simulink library "StateEstimation"  (R2016b)
settings: Solver=VariableStepAuto  StartTime=0.0  StopTime=10.0  RelTol=1e-3
undefined symbols (not defined in the file): accel_bias_init, accel_bias_noise_std, accel_noise_std, cassieParameters, CassieParameters, EKF_SampleTime, gyro_bias_init, gyro_bias_noise_std, gyro_noise_std, q_init, v_init
libraries: xpcutilitieslib x35, xpcrtudplib x35, dspfdesign x10, simulink x6, slrtlib x5
(part 3 of 3)

== system StateEstimation/State Estimator Sim Test/Reconstruct State/Low Pass Filter ==
  signal : Inport  Partition=on  PartitionDimension=1  PartitionWidth=1
  selector : Inport  Port=2
  For Each : ForEach  DisableCoverage=on  IndexMode=One-based
  Lowpass Filter : dspfdesign/Lowpass Filter  FilterType=FIR  DesignForMinimumOrder=on  FilterOrder=50  PassbandFrequency=1  StopbandFrequency=10  PassbandRipple=1  StopbandAttenuation=20  InheritSampleRate=off  SampleRate=2000  SimulateUsing=Code generation  roundingMode=Floor  coeffsDataTypeStr=fixdt(1,16)
  Lowpass Filter1 : dspfdesign/Lowpass Filter  FilterType=FIR  DesignForMinimumOrder=on  FilterOrder=50  PassbandFrequency=1  StopbandFrequency=5  PassbandRipple=1  StopbandAttenuation=30  InheritSampleRate=off  SampleRate=2000  SimulateUsing=Code generation  roundingMode=Floor  coeffsDataTypeStr=fixdt(1,16)
  Switch : Switch  Criteria=u2 > Threshold
  filtered_signal : Outport  ConcatenationDimension=1
  wires:
  signal/1 -> Lowpass Filter1/1, Lowpass Filter/1
  selector/1 -> Switch/2
  Switch/1 -> filtered_signal/1
  Lowpass Filter/1 -> Switch/1
  Lowpass Filter1/1 -> Switch/3

== matlab function StateEstimation/State Estimator/Parse Outputs/Parse_Outputs ==
  data: qwi output; wi output; ai output; q output; outputs input; dq output
function [qwi, wi, ai, q, dq] = Parse_Outputs(outputs)
%
% Frames:
%   W - Cassie World (inertial frame North-West-Up)
%   N - IMU World (inertial frame North-East-Down)
%   B - Body (cassie pelvis)
%   I - IMU (cassie vectorNav)
%   
%   Author: Ross Hartley 
%   Date:   11/06/2017
%

% Parse IMU Data from the VectorNav on Cassie
cassieOutputs = CassieOutputs;
cassieOutputs.setStructure(outputs);

% IMU Data
% VectorNav outputs quaternion as qin = [qw; qx; qy; qz]
qin = cassieOutputs.getVectorNavOrientation; qin = qin([2,3,4,1]); % Convert to [qx; qy; qz; qw] format
wi = cassieOutputs.getVectorNavAngularVelocity;      % {I}_\omega_{NI}   or   {I}_\omega_{WI}
ai = cassieOutputs.getVectorNavLinearAcceleration;   % {I}_a_{NI}        or   {I}_a_{WI}
Rni = Angles.Quaternion_to_Rotation(qin)'; % R_{NI}
Rbi = R_VectorNav_to_Pelvis(zeros(14,1))';    % R_{BI} 
Rwn = Angles.Rx(pi);                % R_{WN}
Rwi = Rwn*Rni;                      % R_{WI}
Rwb = Rwi*Rbi';                     % R_{WB}
qwi = Angles.Rotation_to_Quaternion(Rwi);
 
% Compute angular velocity of body frame:
%      {I}_\omega_{NI} = {I}_\omega_{NW} + {I}_\omega_{WB} + {I}_\omega_{BI}
%                      =        0        + {I}_\omega_{WB} +       0
%  =>  {B}_\omega_{WB} = R_{BI} * {I}_\omega_{NI}
wb = Rbi*wi; % {B}_\omega_{WB}

% Get positions
qq = Angles.Rotation_to_Euler(Rwb);
qaR = cassieOutputs.getRightLegMotorPositions;
qjR =  cassieOutputs.getRightLegJointPositions;
qaL = cassieOutputs.getLeftLegMotorPositions;
qjL =  cassieOutputs.getLeftLegJointPositions;

% Get velocities
dqq = Angles.AngularVelocity_to_EulerRates(qq, wb);
dqaR = cassieOutputs.getRightLegMotorVelocities;
dqjR =  cassieOutputs.getRightLegJointVelocities;
dqaL = cassieOutputs.getLeftLegMotorVelocities;
dqjL =  cassieOutputs.getLeftLegJointVelocities;

% Construct State Vector
q = [zeros(3,1); qq; qaL(1:3); qaL(4); qjL(1); qjL(2); qaL(5); qaR(1:3); qaR(4); qjR(1); qjR(2); qaR(5)];
dq = [zeros(3,1); dqq; dqaL(1:3); dqaL(4); dqjL(1); dqjL(2); dqaL(5); dqaR(1:3); dqaR(4); dqjR(1); dqjR(2); dqaR(5)];

end

== matlab function StateEstimation/State Estimator/Contact Estimator/GRF_Estimator ==
  data: q input; GRF output; contact output
function [GRF, contact] = GRF_Estimator(q)
% Estimates the ground reaction force in the body frame of the robot
%
% Fe_i = (S_i * J_i^T)^{-1} * S_i * \tau_d
%
J_pR = J_RightToeBottom([zeros(6,1); q(7:end)]);
J_pL = J_LeftToeBottom([zeros(6,1); q(7:end)]);

qs_knee_L = q(11);
qs_tarsus_L = q(10) + q(11) + q(12) - deg2rad(13);

qs_knee_R = q(18);
qs_tarsus_R = q(17) + q(18) + q(19) - deg2rad(13);

tau_L = -[1500; 1250].*[qs_knee_L + qs_tarsus_L; qs_tarsus_L];
tau_R = -[1500; 1250].*[qs_knee_R + qs_tarsus_R; qs_tarsus_R];

GRF_L = -[J_pL([1,3],11), J_pL([1,3],12)] \ tau_L;
GRF_R = -[J_pR([1,3],18), J_pR([1,3],19)] \ tau_R;
GRF = [GRF_L; GRF_R];

% Detect contact using GRF
cL = scaleFactor(GRF(2), 50, 100);
cR = scaleFactor(GRF(4), 50, 100);
contact = [cL; cR];

end

== matlab function StateEstimation/Right-Invariant EKF/Contact Estimator/GRF_Estimator ==
  data: q input; GRF output; contact output
function [GRF, contact] = GRF_Estimator(q)
% Estimates the ground reaction force in the body frame of the robot
%
% Fe_i = (S_i * J_i^T)^{-1} * S_i * \tau_d
%
J_pR = J_RightToeBottom([zeros(6,1); q(7:end)]);
J_pL = J_LeftToeBottom([zeros(6,1); q(7:end)]);

qs_knee_L = q(11);
qs_tarsus_L = q(10) + q(11) + q(12) - deg2rad(13);

qs_knee_R = q(18);
qs_tarsus_R = q(17) + q(18) + q(19) - deg2rad(13);

tau_L = -[1500; 1250].*[qs_knee_L + qs_tarsus_L; qs_tarsus_L];
tau_R = -[1500; 1250].*[qs_knee_R + qs_tarsus_R; qs_tarsus_R];

GRF_L = -[J_pL([1,3],11), J_pL([1,3],12)] \ tau_L;
GRF_R = -[J_pR([1,3],18), J_pR([1,3],19)] \ tau_R;
GRF = [GRF_L; GRF_R];

% Detect contact using GRF
cL = scaleFactor(GRF(2), 50, 100);
cR = scaleFactor(GRF(4), 50, 100);
contact = [cL; cR];

end

== matlab function StateEstimation/Right-Invariant EKF/EKF/Send Pose UDP/ConstructPoseData ==
  data: pose_data output; mu input; Sigma input
function pose_data = ConstructPoseData(mu, Sigma)
% Construct pose data for use in ROS network
% Publish everything in pelvis frame
Rwi = Angles.Quaternion_to_Rotation(mu(7:10))';

pose_data = zeros(43,1); 
pose_data(1:3) = mu(1:3) + Rwi*p_VectorNav_to_Pelvis(zeros(14,1));
pose_data(4:7) = Angles.Rotation_to_Quaternion( (Rwi * R_VectorNav_to_Pelvis(zeros(14,1)))' );

% TODO: Convert covariance of IMU pose to Body pose (Ross) 
pose_data(8:end) = reshape(Sigma([1:3,1:3],[7:9,7:9]),[],1);

end

== matlab function StateEstimation/State Estimator/Parse Outputs/Send IMU UDP/Invert Quaterion for ROS ==
  data: q input; q_inv output
function q_inv = fcn(q)
    q_inv = Angles.Rotation_to_Quaternion( Angles.Quaternion_to_Rotation(q)' );
end

== matlab function StateEstimation/Right-Invariant EKF/Kinematic Velocity Estimator/Kinematic_Velocity ==
  data: w input; e input; e_dot input; contact input; velocity output
function velocity  = Kinematic_Velocity(w, e, e_dot, contact)
% Kinematic Velocity Estimator

if contact(1) == 1
    pL = p_VectorNav_to_LeftToeBottom(e); % {I}_p_{IL}
    J_pL = J_VectorNav_to_LeftToeBottom(e);
    velocity = -J_pL(1:3,:)*e_dot - Angles.skew(w)*pL(1:3,:); % {I}_v_{WI}
elseif contact(2) == 1
    pR = p_VectorNav_to_RightToeBottom(e); % {I}_p_{IR}
    J_pR = J_VectorNav_to_RightToeBottom(e);
    velocity = -J_pR(1:3,:)*e_dot - Angles.skew(w)*pR(1:3,:); % {I}_v_{WI}
else
    velocity = zeros(3,1);
end

end

== matlab function StateEstimation/State Estimator/Reconstruct State/Construct_State ==
  data: q output; dq output; q input; dq input; w input; contact input; mu input; ekf_enabled input; velocity output; velocity_kinematic output; filter_selector output
function [q, dq, velocity, velocity_kinematic, filter_selector] = Construct_State(q, dq, w, contact, mu, ekf_enabled)
% Construct state vector and body velocity estimate using raw data and ekf
%   
%   Inputs:
%       q           - state position vector
%       dq          - state velocity vector
%       w           - angular velocity, {I}_\omega_{WI}
%       contact     - contact indicator
%       mu          - EKF state estimate
%       ekf_enabled - EKF enable flag
%
%   Outputs:
%       q                   - 
%       dq                  - 
%       velocity            - EKF body velocity, {W}_v_{WB} 
%       velocity_kinematic  - Kinematic body velocity, {B}_v_{WB} 
%       filter_selector     - used to select low pass filter type
%
%
%   Author: Ross Hartley
%   Date:   11/07/2017

%% Settings
use_ekf_position = true;
use_ekf_orientation = false;
use_ekf_velocity = false;

%% Compute kinematic velocity
e = q(7:end);
e_dot = dq(7:end);

if contact(1) == 1
    pL = p_VectorNav_to_LeftToeBottom(e); % {I}_p_{IL}
    J_pL = J_VectorNav_to_LeftToeBottom(e);
    velocity_kinematic = -J_pL(1:3,:)*e_dot - Angles.skew(w)*pL(1:3,:); % {I}_v_{WI}
elseif contact(2) == 1
    pR = p_VectorNav_to_RightToeBottom(e); % {I}_p_{IR}
    J_pR = J_VectorNav_to_RightToeBottom(e);
    velocity_kinematic = -J_pR(1:3,:)*e_dot - Angles.skew(w)*pR(1:3,:); % {I}_v_{WI}
else
    velocity_kinematic = zeros(3,1);
end

%% Reconstruct State
Rbi = R_VectorNav_to_Pelvis(e)';    % R_{BI}

% Position
if use_ekf_position && ekf_enabled
    Rwi = Angles.Quaternion_to_Rotation(mu(7:10))';
    % {W}_p_{WB} =  {W}_p_{WI} +  {W}_p_{IB}
    q(1:3) = mu(1:3) + Rwi * p_VectorNav_to_Pelvis(e); 
end
 
% Orientation
if use_ekf_orientation && ekf_enabled
    Rwi = Angles.Quaternion_to_Rotation(mu(7:10))';
    Rwb = Rwi * Rbi';
    q(4:6) = Angles.Rotation_to_Euler( Rwb );
end

% Velocity
if use_ekf_velocity && ekf_enabled
    Rwi = Angles.Quaternion_to_Rotation(mu(7:10))';
    Rwb = Rwi * Rbi';
    % {W}_v_{WB} =  {W}_v_{WI} + R_{WI} * skew({I}_w_{WI}) * {I}_p_{IB}
    dq(1:3) = mu(4:6) + Rwi * Angles.skew(w) * p_VectorNav_to_Pelvis(e); 
    % {B}_v_{WB} = R_{BW} * {W}_v_{WB}
    velocity = Rwb' * dq(1:3);
    filter_selector = 1;
else
    Rwb = Angles.Euler_to_Rotation(q(4:6));
    Rwi = Rwb * Rbi;
    % {W}_v_{WB} =  R_{WI} * {I}_v_{WI} + R_{WI} * skew({I}_w_{WI}) * {I}_p_{IB}
    dq(1:3) = Rwi * velocity_kinematic + Rwi * Angles.skew(w) * p_VectorNav_to_Pelvis(e); 
    % {B}_v_{WB} = R_{BW} * {W}_v_{WB}
    velocity = Rwb' * dq(1:3);
    filter_selector = 0;
end



end

== matlab function StateEstimation/State Estimator/Parse Outputs/Send JointState UDP/Parse_Outputs ==
  data: q_reduced output; dq_reduced output; q input; dq input
function [q_reduced, dq_reduced] = ReduceState(q, dq)
% Reduce state vector for use in ROS network

q_reduced = q(7:end);
dq_reduced = dq(7:end);

end

== matlab function StateEstimation/State Estimator/EKF/Send Pose UDP/ConstructPoseData ==
  data: pose_data output; mu input; Sigma input
function pose_data = ConstructPoseData(mu, Sigma)
% Construct pose data for use in ROS network
% Publish everything in pelvis frame
Rwi = Angles.Quaternion_to_Rotation(mu(7:10))';

pose_data = zeros(43,1); 
pose_data(1:3) = mu(1:3) + Rwi*p_VectorNav_to_Pelvis(zeros(14,1));
pose_data(4:7) = Angles.Rotation_to_Quaternion( (Rwi * R_VectorNav_to_Pelvis(zeros(14,1)))' );

% TODO: Convert covariance of IMU pose to Body pose (Ross) 
pose_data(8:end) = reshape(Sigma([1:3,1:3],[7:9,7:9]),[],1);

end

== matlab function StateEstimation/Right-Invariant EKF/Parse Outputs/Parse_Outputs ==
  data: qwi output; wi output; ai output; q output; outputs input; dq output
function [qwi, wi, ai, q, dq] = Parse_Outputs(outputs)
%
% Frames:
%   W - Cassie World (inertial frame North-West-Up)
%   N - IMU World (inertial frame North-East-Down)
%   B - Body (cassie pelvis)
%   I - IMU (cassie vectorNav)
%   
%   Author: Ross Hartley 
%   Date:   11/06/2017
%

% Parse IMU Data from the VectorNav on Cassie
cassieOutputs = CassieOutputs;
cassieOutputs.setStructure(outputs);

% IMU Data
% VectorNav outputs quaternion as qin = [qw; qx; qy; qz]
qin = cassieOutputs.getVectorNavOrientation; qin = qin([2,3,4,1]); % Convert to [qx; qy; qz; qw] format
wi = cassieOutputs.getVectorNavAngularVelocity;      % {I}_\omega_{NI}   or   {I}_\omega_{WI}
ai = cassieOutputs.getVectorNavLinearAcceleration;   % {I}_a_{NI}        or   {I}_a_{WI}
Rni = Angles.Quaternion_to_Rotation(qin)'; % R_{NI}
Rbi = R_VectorNav_to_Pelvis(zeros(14,1))';    % R_{BI} 
Rwn = Angles.Rx(pi);                % R_{WN}
Rwi = Rwn*Rni;                      % R_{WI}
Rwb = Rwi*Rbi';                     % R_{WB}
qwi = Angles.Rotation_to_Quaternion(Rwi);
 
% Compute angular velocity of body frame:
%      {I}_\omega_{NI} = {I}_\omega_{NW} + {I}_\omega_{WB} + {I}_\omega_{BI}
%                      =        0        + {I}_\omega_{WB} +       0
%  =>  {B}_\omega_{WB} = R_{BI} * {I}_\omega_{NI}
wb = Rbi*wi; % {B}_\omega_{WB}

% Get positions
qq = Angles.Rotation_to_Euler(Rwb);
qaR = cassieOutputs.getRightLegMotorPositions;
qjR =  cassieOutputs.getRightLegJointPositions;
qaL = cassieOutputs.getLeftLegMotorPositions;
qjL =  cassieOutputs.getLeftLegJointPositions;

% Get velocities
dqq = Angles.AngularVelocity_to_EulerRates(qq, wb);
dqaR = cassieOutputs.getRightLegMotorVelocities;
dqjR =  cassieOutputs.getRightLegJointVelocities;
dqaL = cassieOutputs.getLeftLegMotorVelocities;
dqjL =  cassieOutputs.getLeftLegJointVelocities;

% Construct State Vector
q = [zeros(3,1); qq; qaL(1:3); qaL(4); qjL(1); qjL(2); qaL(5); qaR(1:3); qaR(4); qjR(1); qjR(2); qaR(5)];
dq = [zeros(3,1); dqq; dqaL(1:3); dqaL(4); dqjL(1); dqjL(2); dqaL(5); dqaR(1:3); dqaR(4); dqjR(1); dqjR(2); dqaR(5)];

end

== matlab function StateEstimation/State Estimator Sim Test/Contact Estimator/GRF_Estimator ==
  data: q input; GRF output; contact output
function [GRF, contact] = GRF_Estimator(q)
% Estimates the ground reaction force in the body frame of the robot
%
% Fe_i = (S_i * J_i^T)^{-1} * S_i * \tau_d
%
J_pR = J_RightToeBottom([zeros(6,1); q(7:end)]);
J_pL = J_LeftToeBottom([zeros(6,1); q(7:end)]);

qs_knee_L = q(11);
qs_tarsus_L = q(10) + q(11) + q(12) - deg2rad(13);

qs_knee_R = q(18);
qs_tarsus_R = q(17) + q(18) + q(19) - deg2rad(13);

tau_L = -[1500; 1250].*[qs_knee_L + qs_tarsus_L; qs_tarsus_L];
tau_R = -[1500; 1250].*[qs_knee_R + qs_tarsus_R; qs_tarsus_R];

GRF_L = -[J_pL([1,3],11), J_pL([1,3],12)] \ tau_L;
GRF_R = -[J_pR([1,3],18), J_pR([1,3],19)] \ tau_R;
GRF = [GRF_L; GRF_R];

% Detect contact using GRF
cL = scaleFactor(GRF(2), 50, 100);
cR = scaleFactor(GRF(4), 50, 100);
contact = [cL; cR];

end

== matlab function StateEstimation/Right-Invariant EKF/Parse Outputs/Send IMU UDP/Invert Quaterion for ROS ==
  data: q input; q_inv output
function q_inv = fcn(q)
    q_inv = Angles.Rotation_to_Quaternion( Angles.Quaternion_to_Rotation(q)' );
end

== matlab function StateEstimation/Right-Invariant EKF/Parse Outputs/Send JointState UDP/Parse_Outputs ==
  data: q_reduced output; dq_reduced output; q input; dq input
function [q_reduced, dq_reduced] = ReduceState(q, dq)
% Reduce state vector for use in ROS network

q_reduced = q(7:end);
dq_reduced = dq(7:end);

end

== matlab function StateEstimation/State Estimator Sim Test/EKF/Send Pose UDP/ConstructPoseData ==
  data: pose_data output; mu input; Sigma input
function pose_data = ConstructPoseData(mu, Sigma)
% Construct pose data for use in ROS network
% Publish everything in pelvis frame
Rwi = Angles.Quaternion_to_Rotation(mu(7:10))';

pose_data = zeros(43,1); 
pose_data(1:3) = mu(1:3) + Rwi*p_VectorNav_to_Pelvis(zeros(14,1));
pose_data(4:7) = Angles.Rotation_to_Quaternion( (Rwi * R_VectorNav_to_Pelvis(zeros(14,1)))' );

% TODO: Convert covariance of IMU pose to Body pose (Ross) 
pose_data(8:end) = reshape(Sigma([1:3,1:3],[7:9,7:9]),[],1);

end

== matlab function StateEstimation/State Estimator Sim Test/Kinematic Velocity Estimator/Kinematic_Velocity ==
  data: w input; e input; e_dot input; contact input; velocity output
function velocity  = Kinematic_Velocity(w, e, e_dot, contact)
% Kinematic Velocity Estimator

if contact(1) == 1
    pL = p_VectorNav_to_LeftToeBottom(e); % {I}_p_{IL}
    J_pL = J_VectorNav_to_LeftToeBottom(e);
    velocity = -J_pL(1:3,:)*e_dot - Angles.skew(w)*pL(1:3,:); % {I}_v_{WI}
elseif contact(2) == 1
    pR = p_VectorNav_to_RightToeBottom(e); % {I}_p_{IR}
    J_pR = J_VectorNav_to_RightToeBottom(e);
    velocity = -J_pR(1:3,:)*e_dot - Angles.skew(w)*pR(1:3,:); % {I}_v_{WI}
else
    velocity = zeros(3,1);
end

end

== matlab function StateEstimation/State Estimator Sim Test/Parse Outputs/Parse_Outputs ==
  data: qwi output; wi output; ai output; q output; outputs input; dq output
function [qwi, wi, ai, q, dq] = Parse_Outputs(outputs)
%
% Frames:
%   W - Cassie World (inertial frame North-West-Up)
%   N - IMU World (inertial frame North-East-Down)
%   B - Body (cassie pelvis)
%   I - IMU (cassie vectorNav)
%   
%   Author: Ross Hartley 
%   Date:   11/06/2017
%

% Parse IMU Data from the VectorNav on Cassie
cassieOutputs = CassieOutputs;
cassieOutputs.setStructure(outputs);

% IMU Data
% VectorNav outputs quaternion as qin = [qw; qx; qy; qz]
qin = cassieOutputs.getVectorNavOrientation; qin = qin([2,3,4,1]); % Convert to [qx; qy; qz; qw] format
wi = cassieOutputs.getVectorNavAngularVelocity;      % {I}_\omega_{NI}   or   {I}_\omega_{WI}
ai = cassieOutputs.getVectorNavLinearAcceleration;   % {I}_a_{NI}        or   {I}_a_{WI}
Rni = Angles.Quaternion_to_Rotation(qin)'; % R_{NI}
Rbi = R_VectorNav_to_Pelvis(zeros(14,1))';    % R_{BI} 
Rwn = Angles.Rx(pi);                % R_{WN}
Rwi = Rwn*Rni;                      % R_{WI}
Rwb = Rwi*Rbi';                     % R_{WB}
qwi = Angles.Rotation_to_Quaternion(Rwi);
 
% Compute angular velocity of body frame:
%      {I}_\omega_{NI} = {I}_\omega_{NW} + {I}_\omega_{WB} + {I}_\omega_{BI}
%                      =        0        + {I}_\omega_{WB} +       0
%  =>  {B}_\omega_{WB} = R_{BI} * {I}_\omega_{NI}
wb = Rbi*wi; % {B}_\omega_{WB}

% Get positions
qq = Angles.Rotation_to_Euler(Rwb);
qaR = cassieOutputs.getRightLegMotorPositions;
qjR =  cassieOutputs.getRightLegJointPositions;
qaL = cassieOutputs.getLeftLegMotorPositions;
qjL =  cassieOutputs.getLeftLegJointPositions;

% Get velocities
dqq = Angles.AngularVelocity_to_EulerRates(qq, wb);
dqaR = cassieOutputs.getRightLegMotorVelocities;
dqjR =  cassieOutputs.getRightLegJointVelocities;
dqaL = cassieOutputs.getLeftLegMotorVelocities;
dqjL =  cassieOutputs.getLeftLegJointVelocities;

% Construct State Vector
q = [zeros(3,1); qq; qaL(1:3); qaL(4); qjL(1); qjL(2); qaL(5); qaR(1:3); qaR(4); qjR(1); qjR(2); qaR(5)];
dq = [zeros(3,1); dqq; dqaL(1:3); dqaL(4); dqjL(1); dqjL(2); dqaL(5); dqaR(1:3); dqaR(4); dqjR(1); dqjR(2); dqaR(5)];

end

== matlab function StateEstimation/State Estimator Sim Test/Parse Outputs/Send IMU UDP/Invert Quaterion for ROS ==
  data: q input; q_inv output
function q_inv = fcn(q)
    q_inv = Angles.Rotation_to_Quaternion( Angles.Quaternion_to_Rotation(q)' );
end

== matlab function StateEstimation/State Estimator Sim Test/Parse Outputs/Send JointState UDP/Parse_Outputs ==
  data: q_reduced output; dq_reduced output; q input; dq input
function [q_reduced, dq_reduced] = ReduceState(q, dq)
% Reduce state vector for use in ROS network

q_reduced = q(7:end);
dq_reduced = dq(7:end);

end

== matlab function StateEstimation/State Estimator/Kinematic Velocity Estimator/Kinematic_Velocity ==
  data: w input; e input; e_dot input; contact input; velocity output
function velocity  = Kinematic_Velocity(w, e, e_dot, contact)
% Kinematic Velocity Estimator

if contact(1) == 1
    pL = p_VectorNav_to_LeftToeBottom(e); % {I}_p_{IL}
    J_pL = J_VectorNav_to_LeftToeBottom(e);
    velocity = -J_pL(1:3,:)*e_dot - Angles.skew(w)*pL(1:3,:); % {I}_v_{WI}
elseif contact(2) == 1
    pR = p_VectorNav_to_RightToeBottom(e); % {I}_p_{IR}
    J_pR = J_VectorNav_to_RightToeBottom(e);
    velocity = -J_pR(1:3,:)*e_dot - Angles.skew(w)*pR(1:3,:); % {I}_v_{WI}
else
    velocity = zeros(3,1);
end

end

== matlab function StateEstimation/State Estimator Sim Test/Reconstruct State/Construct_State ==
  data: q output; dq output; q input; dq input; w input; contact input; mu input; ekf_enabled input; velocity output; velocity_kinematic output; filter_selector output
function [q, dq, velocity, velocity_kinematic, filter_selector] = Construct_State(q, dq, w, contact, mu, ekf_enabled)
% Construct state vector and body velocity estimate using raw data and ekf
%   
%   Inputs:
%       q           - state position vector
%       dq          - state velocity vector
%       w           - angular velocity, {I}_\omega_{WI}
%       contact     - contact indicator
%       mu          - EKF state estimate
%       ekf_enabled - EKF enable flag
%
%   Outputs:
%       q                   - 
%       dq                  - 
%       velocity            - EKF body velocity, {W}_v_{WB} 
%       velocity_kinematic  - Kinematic body velocity, {B}_v_{WB} 
%       filter_selector     - used to select low pass filter type
%
%
%   Author: Ross Hartley
%   Date:   11/07/2017

%% Settings
use_ekf_position = true;
use_ekf_orientation = false;
use_ekf_velocity = false;

%% Compute kinematic velocity
e = q(7:end);
e_dot = dq(7:end);

if contact(1) == 1
    pL = p_VectorNav_to_LeftToeBottom(e); % {I}_p_{IL}
    J_pL = J_VectorNav_to_LeftToeBottom(e);
    velocity_kinematic = -J_pL(1:3,:)*e_dot - Angles.skew(w)*pL(1:3,:); % {I}_v_{WI}
elseif contact(2) == 1
    pR = p_VectorNav_to_RightToeBottom(e); % {I}_p_{IR}
    J_pR = J_VectorNav_to_RightToeBottom(e);
    velocity_kinematic = -J_pR(1:3,:)*e_dot - Angles.skew(w)*pR(1:3,:); % {I}_v_{WI}
else
    velocity_kinematic = zeros(3,1);
end

%% Reconstruct State
Rbi = R_VectorNav_to_Pelvis(e)';    % R_{BI}

% Position
if use_ekf_position && ekf_enabled
    Rwi = Angles.Quaternion_to_Rotation(mu(7:10))';
    % {W}_p_{WB} =  {W}_p_{WI} +  {W}_p_{IB}
    q(1:3) = mu(1:3) + Rwi * p_VectorNav_to_Pelvis(e); 
end
 
% Orientation
if use_ekf_orientation && ekf_enabled
    Rwi = Angles.Quaternion_to_Rotation(mu(7:10))';
    Rwb = Rwi * Rbi';
    q(4:6) = Angles.Rotation_to_Euler( Rwb );
end

% Velocity
if use_ekf_velocity && ekf_enabled
    Rwi = Angles.Quaternion_to_Rotation(mu(7:10))';
    Rwb = Rwi * Rbi';
    % {W}_v_{WB} =  {W}_v_{WI} + R_{WI} * skew({I}_w_{WI}) * {I}_p_{IB}
    dq(1:3) = mu(4:6) + Rwi * Angles.skew(w) * p_VectorNav_to_Pelvis(e); 
    % {B}_v_{WB} = R_{BW} * {W}_v_{WB}
    velocity = Rwb' * dq(1:3);
    filter_selector = 1;
else
    Rwb = Angles.Euler_to_Rotation(q(4:6));
    Rwi = Rwb * Rbi;
    % {W}_v_{WB} =  R_{WI} * {I}_v_{WI} + R_{WI} * skew({I}_w_{WI}) * {I}_p_{IB}
    dq(1:3) = Rwi * velocity_kinematic + Rwi * Angles.skew(w) * p_VectorNav_to_Pelvis(e); 
    % {B}_v_{WB} = R_{BW} * {W}_v_{WB}
    velocity = Rwb' * dq(1:3);
    filter_selector = 0;
end



end

== matlab function StateEstimation/Kinematic Velocity Estimator/Kinematic_Velocity ==
  data: w input; e input; e_dot input; contact input; velocity output
function velocity  = Kinematic_Velocity(w, e, e_dot, contact)
% Kinematic Velocity Estimator

if contact(1) == 1
    pL = p_VectorNav_to_LeftToeBottom(e); % {I}_p_{IL}
    J_pL = J_VectorNav_to_LeftToeBottom(e);
    velocity = -J_pL(1:3,:)*e_dot - Angles.skew(w)*pL(1:3,:); % {I}_v_{WI}
elseif contact(2) == 1
    pR = p_VectorNav_to_RightToeBottom(e); % {I}_p_{IR}
    J_pR = J_VectorNav_to_RightToeBottom(e);
    velocity = -J_pR(1:3,:)*e_dot - Angles.skew(w)*pR(1:3,:); % {I}_v_{WI}
else
    velocity = zeros(3,1);
end

end

== matlab function StateEstimation/State Estimator Exp Test/Contact Estimator/GRF_Estimator ==
  data: q input; GRF output; contact output
function [GRF, contact] = GRF_Estimator(q)
% Estimates the ground reaction force in the body frame of the robot
%
% Fe_i = (S_i * J_i^T)^{-1} * S_i * \tau_d
%
J_pR = J_RightToeBottom([zeros(6,1); q(7:end)]);
J_pL = J_LeftToeBottom([zeros(6,1); q(7:end)]);

qs_knee_L = q(11);
qs_tarsus_L = q(10) + q(11) + q(12) - deg2rad(13);

qs_knee_R = q(18);
qs_tarsus_R = q(17) + q(18) + q(19) - deg2rad(13);

tau_L = -[1500; 1250].*[qs_knee_L + qs_tarsus_L; qs_tarsus_L];
tau_R = -[1500; 1250].*[qs_knee_R + qs_tarsus_R; qs_tarsus_R];

GRF_L = -[J_pL([1,3],11), J_pL([1,3],12)] \ tau_L;
GRF_R = -[J_pR([1,3],18), J_pR([1,3],19)] \ tau_R;
GRF = [GRF_L; GRF_R];

% Detect contact using GRF
cL = scaleFactor(GRF(2), 50, 100);
cR = scaleFactor(GRF(4), 50, 100);
contact = [cL; cR];

end

== matlab function StateEstimation/State Estimator Exp Test/EKF/Send Pose UDP/ConstructPoseData ==
  data: pose_data output; mu input; Sigma input
function pose_data = ConstructPoseData(mu, Sigma)
% Construct pose data for use in ROS network
% Publish everything in pelvis frame
Rwi = Angles.Quaternion_to_Rotation(mu(7:10))';

pose_data = zeros(43,1); 
pose_data(1:3) = mu(1:3) + Rwi*p_VectorNav_to_Pelvis(zeros(14,1));
pose_data(4:7) = Angles.Rotation_to_Quaternion( (Rwi * R_VectorNav_to_Pelvis(zeros(14,1)))' );

% TODO: Convert covariance of IMU pose to Body pose (Ross) 
pose_data(8:end) = reshape(Sigma([1:3,1:3],[7:9,7:9]),[],1);

end

== matlab function StateEstimation/State Estimator Exp Test/Kinematic Velocity Estimator/Kinematic_Velocity ==
  data: w input; e input; e_dot input; contact input; velocity output
function velocity  = Kinematic_Velocity(w, e, e_dot, contact)
% Kinematic Velocity Estimator

if contact(1) == 1
    pL = p_VectorNav_to_LeftToeBottom(e); % {I}_p_{IL}
    J_pL = J_VectorNav_to_LeftToeBottom(e);
    velocity = -J_pL(1:3,:)*e_dot - Angles.skew(w)*pL(1:3,:); % {I}_v_{WI}
elseif contact(2) == 1
    pR = p_VectorNav_to_RightToeBottom(e); % {I}_p_{IR}
    J_pR = J_VectorNav_to_RightToeBottom(e);
    velocity = -J_pR(1:3,:)*e_dot - Angles.skew(w)*pR(1:3,:); % {I}_v_{WI}
else
    velocity = zeros(3,1);
end

end

== matlab function StateEstimation/State Estimator Exp Test/Parse Outputs/Parse_Outputs ==
  data: qwi output; wi output; ai output; q output; outputs input; dq output
function [qwi, wi, ai, q, dq] = Parse_Outputs(outputs)
%
% Frames:
%   W - Cassie World (inertial frame North-West-Up)
%   N - IMU World (inertial frame North-East-Down)
%   B - Body (cassie pelvis)
%   I - IMU (cassie vectorNav)
%   
%   Author: Ross Hartley 
%   Date:   11/06/2017
%

% Parse IMU Data from the VectorNav on Cassie
cassieOutputs = CassieOutputs;
cassieOutputs.setStructure(outputs);

% IMU Data
% VectorNav outputs quaternion as qin = [qw; qx; qy; qz]
qin = cassieOutputs.getVectorNavOrientation; qin = qin([2,3,4,1]); % Convert to [qx; qy; qz; qw] format
wi = cassieOutputs.getVectorNavAngularVelocity;      % {I}_\omega_{NI}   or   {I}_\omega_{WI}
ai = cassieOutputs.getVectorNavLinearAcceleration;   % {I}_a_{NI}        or   {I}_a_{WI}
Rni = Angles.Quaternion_to_Rotation(qin)'; % R_{NI}
Rbi = R_VectorNav_to_Pelvis(zeros(14,1))';    % R_{BI} 
Rwn = Angles.Rx(pi);                % R_{WN}
Rwi = Rwn*Rni;                      % R_{WI}
Rwb = Rwi*Rbi';                     % R_{WB}
qwi = Angles.Rotation_to_Quaternion(Rwi);
 
% Compute angular velocity of body frame:
%      {I}_\omega_{NI} = {I}_\omega_{NW} + {I}_\omega_{WB} + {I}_\omega_{BI}
%                      =        0        + {I}_\omega_{WB} +       0
%  =>  {B}_\omega_{WB} = R_{BI} * {I}_\omega_{NI}
wb = Rbi*wi; % {B}_\omega_{WB}

% Get positions
qq = Angles.Rotation_to_Euler(Rwb);
qaR = cassieOutputs.getRightLegMotorPositions;
qjR =  cassieOutputs.getRightLegJointPositions;
qaL = cassieOutputs.getLeftLegMotorPositions;
qjL =  cassieOutputs.getLeftLegJointPositions;

% Get velocities
dqq = Angles.AngularVelocity_to_EulerRates(qq, wb);
dqaR = cassieOutputs.getRightLegMotorVelocities;
dqjR =  cassieOutputs.getRightLegJointVelocities;
dqaL = cassieOutputs.getLeftLegMotorVelocities;
dqjL =  cassieOutputs.getLeftLegJointVelocities;

% Construct State Vector
q = [zeros(3,1); qq; qaL(1:3); qaL(4); qjL(1); qjL(2); qaL(5); qaR(1:3); qaR(4); qjR(1); qjR(2); qaR(5)];
dq = [zeros(3,1); dqq; dqaL(1:3); dqaL(4); dqjL(1); dqjL(2); dqaL(5); dqaR(1:3); dqaR(4); dqjR(1); dqjR(2); dqaR(5)];

end

== matlab function StateEstimation/State Estimator Exp Test/Parse Outputs/Send IMU UDP/Invert Quaterion for ROS ==
  data: q input; q_inv output
function q_inv = fcn(q)
    q_inv = Angles.Rotation_to_Quaternion( Angles.Quaternion_to_Rotation(q)' );
end

== matlab function StateEstimation/State Estimator Exp Test/Parse Outputs/Send JointState UDP/Parse_Outputs ==
  data: q_reduced output; dq_reduced output; q input; dq input
function [q_reduced, dq_reduced] = ReduceState(q, dq)
% Reduce state vector for use in ROS network

q_reduced = q(7:end);
dq_reduced = dq(7:end);

end

== matlab function StateEstimation/State Estimator Exp Test/Reconstruct State/Construct_State ==
  data: q output; dq output; q input; dq input; w input; contact input; mu input; ekf_enabled input; velocity output; velocity_kinematic output; filter_selector output
function [q, dq, velocity, velocity_kinematic, filter_selector] = Construct_State(q, dq, w, contact, mu, ekf_enabled)
% Construct state vector and body velocity estimate using raw data and ekf
%   
%   Inputs:
%       q           - state position vector
%       dq          - state velocity vector
%       w           - angular velocity, {I}_\omega_{WI}
%       contact     - contact indicator
%       mu          - EKF state estimate
%       ekf_enabled - EKF enable flag
%
%   Outputs:
%       q                   - 
%       dq                  - 
%       velocity            - EKF body velocity, {W}_v_{WB} 
%       velocity_kinematic  - Kinematic body velocity, {B}_v_{WB} 
%       filter_selector     - used to select low pass filter type
%
%
%   Author: Ross Hartley
%   Date:   11/07/2017

%% Settings
use_ekf_position = true;
use_ekf_orientation = false;
use_ekf_velocity = false;

%% Compute kinematic velocity
e = q(7:end);
e_dot = dq(7:end);

if contact(1) == 1
    pL = p_VectorNav_to_LeftToeBottom(e); % {I}_p_{IL}
    J_pL = J_VectorNav_to_LeftToeBottom(e);
    velocity_kinematic = -J_pL(1:3,:)*e_dot - Angles.skew(w)*pL(1:3,:); % {I}_v_{WI}
elseif contact(2) == 1
    pR = p_VectorNav_to_RightToeBottom(e); % {I}_p_{IR}
    J_pR = J_VectorNav_to_RightToeBottom(e);
    velocity_kinematic = -J_pR(1:3,:)*e_dot - Angles.skew(w)*pR(1:3,:); % {I}_v_{WI}
else
    velocity_kinematic = zeros(3,1);
end

%% Reconstruct State
Rbi = R_VectorNav_to_Pelvis(e)';    % R_{BI}

% Position
if use_ekf_position && ekf_enabled
    Rwi = Angles.Quaternion_to_Rotation(mu(7:10))';
    % {W}_p_{WB} =  {W}_p_{WI} +  {W}_p_{IB}
    q(1:3) = mu(1:3) + Rwi * p_VectorNav_to_Pelvis(e); 
end
 
% Orientation
if use_ekf_orientation && ekf_enabled
    Rwi = Angles.Quaternion_to_Rotation(mu(7:10))';
    Rwb = Rwi * Rbi';
    q(4:6) = Angles.Rotation_to_Euler( Rwb );
end

% Velocity
if use_ekf_velocity && ekf_enabled
    Rwi = Angles.Quaternion_to_Rotation(mu(7:10))';
    Rwb = Rwi * Rbi';
    % {W}_v_{WB} =  {W}_v_{WI} + R_{WI} * skew({I}_w_{WI}) * {I}_p_{IB}
    dq(1:3) = mu(4:6) + Rwi * Angles.skew(w) * p_VectorNav_to_Pelvis(e); 
    % {B}_v_{WB} = R_{BW} * {W}_v_{WB}
    velocity = Rwb' * dq(1:3);
    filter_selector = 1;
else
    Rwb = Angles.Euler_to_Rotation(q(4:6));
    Rwi = Rwb * Rbi;
    % {W}_v_{WB} =  R_{WI} * {I}_v_{WI} + R_{WI} * skew({I}_w_{WI}) * {I}_p_{IB}
    dq(1:3) = Rwi * velocity_kinematic + Rwi * Angles.skew(w) * p_VectorNav_to_Pelvis(e); 
    % {B}_v_{WB} = R_{BW} * {W}_v_{WB}
    velocity = Rwb' * dq(1:3);
    filter_selector = 0;
end



end

== matlab function StateEstimation/Right-Invariant EKF/Reconstruct State/Construct_State ==
  data: q output; dq output; q input; dq input; w input; contact input; mu input; ekf_enabled input; velocity output; velocity_kinematic output; filter_selector output
function [q, dq, velocity, velocity_kinematic, filter_selector] = Construct_State(q, dq, w, contact, mu, ekf_enabled)
% Construct state vector and body velocity estimate using raw data and ekf
%   
%   Inputs:
%       q           - state position vector
%       dq          - state velocity vector
%       w           - angular velocity, {I}_\omega_{WI}
%       contact     - contact indicator
%       mu          - EKF state estimate
%       ekf_enabled - EKF enable flag
%
%   Outputs:
%       q                   - 
%       dq                  - 
%       velocity            - EKF body velocity, {W}_v_{WB} 
%       velocity_kinematic  - Kinematic body velocity, {B}_v_{WB} 
%       filter_selector     - used to select low pass filter type
%
%
%   Author: Ross Hartley
%   Date:   11/07/2017

%% Settings
use_ekf_position = true;
use_ekf_orientation = false;
use_ekf_velocity = false;

%% Compute kinematic velocity
e = q(7:end);
e_dot = dq(7:end);

if contact(1) == 1
    pL = p_VectorNav_to_LeftToeBottom(e); % {I}_p_{IL}
    J_pL = J_VectorNav_to_LeftToeBottom(e);
    velocity_kinematic = -J_pL(1:3,:)*e_dot - Angles.skew(w)*pL(1:3,:); % {I}_v_{WI}
elseif contact(2) == 1
    pR = p_VectorNav_to_RightToeBottom(e); % {I}_p_{IR}
    J_pR = J_VectorNav_to_RightToeBottom(e);
    velocity_kinematic = -J_pR(1:3,:)*e_dot - Angles.skew(w)*pR(1:3,:); % {I}_v_{WI}
else
    velocity_kinematic = zeros(3,1);
end

%% Reconstruct State
Rbi = R_VectorNav_to_Pelvis(e)';    % R_{BI}

% Position
if use_ekf_position && ekf_enabled
    Rwi = Angles.Quaternion_to_Rotation(mu(7:10))';
    % {W}_p_{WB} =  {W}_p_{WI} +  {W}_p_{IB}
    q(1:3) = mu(1:3) + Rwi * p_VectorNav_to_Pelvis(e); 
end
 
% Orientation
if use_ekf_orientation && ekf_enabled
    Rwi = Angles.Quaternion_to_Rotation(mu(7:10))';
    Rwb = Rwi * Rbi';
    q(4:6) = Angles.Rotation_to_Euler( Rwb );
end

% Velocity
if use_ekf_velocity && ekf_enabled
    Rwi = Angles.Quaternion_to_Rotation(mu(7:10))';
    Rwb = Rwi * Rbi';
    % {W}_v_{WB} =  {W}_v_{WI} + R_{WI} * skew({I}_w_{WI}) * {I}_p_{IB}
    dq(1:3) = mu(4:6) + Rwi * Angles.skew(w) * p_VectorNav_to_Pelvis(e); 
    % {B}_v_{WB} = R_{BW} * {W}_v_{WB}
    velocity = Rwb' * dq(1:3);
    filter_selector = 1;
else
    Rwb = Angles.Euler_to_Rotation(q(4:6));
    Rwi = Rwb * Rbi;
    % {W}_v_{WB} =  R_{WI} * {I}_v_{WI} + R_{WI} * skew({I}_w_{WI}) * {I}_p_{IB}
    dq(1:3) = Rwi * velocity_kinematic + Rwi * Angles.skew(w) * p_VectorNav_to_Pelvis(e); 
    % {B}_v_{WB} = R_{BW} * {W}_v_{WB}
    velocity = Rwb' * dq(1:3);
    filter_selector = 0;
end



end

== matlab function StateEstimation/Quaternion-based EKF/Contact Estimator/GRF_Estimator ==
  data: q input; GRF output; contact output
function [GRF, contact] = GRF_Estimator(q)
% Estimates the ground reaction force in the body frame of the robot
%
% Fe_i = (S_i * J_i^T)^{-1} * S_i * \tau_d
%
J_pR = J_RightToeBottom([zeros(6,1); q(7:end)]);
J_pL = J_LeftToeBottom([zeros(6,1); q(7:end)]);

qs_knee_L = q(11);
qs_tarsus_L = q(10) + q(11) + q(12) - deg2rad(13);

qs_knee_R = q(18);
qs_tarsus_R = q(17) + q(18) + q(19) - deg2rad(13);

tau_L = -[1500; 1250].*[qs_knee_L + qs_tarsus_L; qs_tarsus_L];
tau_R = -[1500; 1250].*[qs_knee_R + qs_tarsus_R; qs_tarsus_R];

GRF_L = -[J_pL([1,3],11), J_pL([1,3],12)] \ tau_L;
GRF_R = -[J_pR([1,3],18), J_pR([1,3],19)] \ tau_R;
GRF = [GRF_L; GRF_R];

% Detect contact using GRF
cL = scaleFactor(GRF(2), 50, 100);
cR = scaleFactor(GRF(4), 50, 100);
contact = [cL; cR];

end

== matlab function StateEstimation/Quaternion-based EKF/EKF/Send Pose UDP/ConstructPoseData ==
  data: pose_data output; mu input; Sigma input
function pose_data = ConstructPoseData(mu, Sigma)
% Construct pose data for use in ROS network
% Publish everything in pelvis frame
Rwi = Angles.Quaternion_to_Rotation(mu(7:10))';

pose_data = zeros(43,1); 
pose_data(1:3) = mu(1:3) + Rwi*p_VectorNav_to_Pelvis(zeros(14,1));
pose_data(4:7) = Angles.Rotation_to_Quaternion( (Rwi * R_VectorNav_to_Pelvis(zeros(14,1)))' );

% TODO: Convert covariance of IMU pose to Body pose (Ross) 
pose_data(8:end) = reshape(Sigma([1:3,1:3],[7:9,7:9]),[],1);

end

== matlab function StateEstimation/Quaternion-based EKF/Kinematic Velocity Estimator/Kinematic_Velocity ==
  data: w input; e input; e_dot input; contact input; velocity output
function velocity  = Kinematic_Velocity(w, e, e_dot, contact)
% Kinematic Velocity Estimator

if contact(1) == 1
    pL = p_VectorNav_to_LeftToeBottom(e); % {I}_p_{IL}
    J_pL = J_VectorNav_to_LeftToeBottom(e);
    velocity = -J_pL(1:3,:)*e_dot - Angles.skew(w)*pL(1:3,:); % {I}_v_{WI}
elseif contact(2) == 1
    pR = p_VectorNav_to_RightToeBottom(e); % {I}_p_{IR}
    J_pR = J_VectorNav_to_RightToeBottom(e);
    velocity = -J_pR(1:3,:)*e_dot - Angles.skew(w)*pR(1:3,:); % {I}_v_{WI}
else
    velocity = zeros(3,1);
end

end

== matlab function StateEstimation/Quaternion-based EKF/Parse Outputs/Parse_Outputs ==
  data: qwi output; wi output; ai output; q output; outputs input; dq output
function [qwi, wi, ai, q, dq] = Parse_Outputs(outputs)
%
% Frames:
%   W - Cassie World (inertial frame North-West-Up)
%   N - IMU World (inertial frame North-East-Down)
%   B - Body (cassie pelvis)
%   I - IMU (cassie vectorNav)
%   
%   Author: Ross Hartley 
%   Date:   11/06/2017
%

% Parse IMU Data from the VectorNav on Cassie
cassieOutputs = CassieOutputs;
cassieOutputs.setStructure(outputs);

% IMU Data
% VectorNav outputs quaternion as qin = [qw; qx; qy; qz]
qin = cassieOutputs.getVectorNavOrientation; qin = qin([2,3,4,1]); % Convert to [qx; qy; qz; qw] format
wi = cassieOutputs.getVectorNavAngularVelocity;      % {I}_\omega_{NI}   or   {I}_\omega_{WI}
ai = cassieOutputs.getVectorNavLinearAcceleration;   % {I}_a_{NI}        or   {I}_a_{WI}
Rni = Angles.Quaternion_to_Rotation(qin)'; % R_{NI}
Rbi = R_VectorNav_to_Pelvis(zeros(14,1))';    % R_{BI} 
Rwn = Angles.Rx(pi);                % R_{WN}
Rwi = Rwn*Rni;                      % R_{WI}
Rwb = Rwi*Rbi';                     % R_{WB}
qwi = Angles.Rotation_to_Quaternion(Rwi);
 
% Compute angular velocity of body frame:
%      {I}_\omega_{NI} = {I}_\omega_{NW} + {I}_\omega_{WB} + {I}_\omega_{BI}
%                      =        0        + {I}_\omega_{WB} +       0
%  =>  {B}_\omega_{WB} = R_{BI} * {I}_\omega_{NI}
wb = Rbi*wi; % {B}_\omega_{WB}

% Get positions
qq = Angles.Rotation_to_Euler(Rwb);
qaR = cassieOutputs.getRightLegMotorPositions;
qjR =  cassieOutputs.getRightLegJointPositions;
qaL = cassieOutputs.getLeftLegMotorPositions;
qjL =  cassieOutputs.getLeftLegJointPositions;

% Get velocities
dqq = Angles.AngularVelocity_to_EulerRates(qq, wb);
dqaR = cassieOutputs.getRightLegMotorVelocities;
dqjR =  cassieOutputs.getRightLegJointVelocities;
dqaL = cassieOutputs.getLeftLegMotorVelocities;
dqjL =  cassieOutputs.getLeftLegJointVelocities;

% Construct State Vector
q = [zeros(3,1); qq; qaL(1:3); qaL(4); qjL(1); qjL(2); qaL(5); qaR(1:3); qaR(4); qjR(1); qjR(2); qaR(5)];
dq = [zeros(3,1); dqq; dqaL(1:3); dqaL(4); dqjL(1); dqjL(2); dqaL(5); dqaR(1:3); dqaR(4); dqjR(1); dqjR(2); dqaR(5)];

end

== matlab function StateEstimation/Quaternion-based EKF/Parse Outputs/Send IMU UDP/Invert Quaterion for ROS ==
  data: q input; q_inv output
function q_inv = fcn(q)
    q_inv = Angles.Rotation_to_Quaternion( Angles.Quaternion_to_Rotation(q)' );
end

== matlab function StateEstimation/Quaternion-based EKF/Parse Outputs/Send JointState UDP/Parse_Outputs ==
  data: q_reduced output; dq_reduced output; q input; dq input
function [q_reduced, dq_reduced] = ReduceState(q, dq)
% Reduce state vector for use in ROS network

q_reduced = q(7:end);
dq_reduced = dq(7:end);

end

== matlab function StateEstimation/Quaternion-based EKF/Reconstruct State/Construct_State ==
  data: q output; dq output; q input; dq input; w input; contact input; mu input; ekf_enabled input; velocity output; velocity_kinematic output; filter_selector output
function [q, dq, velocity, velocity_kinematic, filter_selector] = Construct_State(q, dq, w, contact, mu, ekf_enabled)
% Construct state vector and body velocity estimate using raw data and ekf
%   
%   Inputs:
%       q           - state position vector
%       dq          - state velocity vector
%       w           - angular velocity, {I}_\omega_{WI}
%       contact     - contact indicator
%       mu          - EKF state estimate
%       ekf_enabled - EKF enable flag
%
%   Outputs:
%       q                   - 
%       dq                  - 
%       velocity            - EKF body velocity, {W}_v_{WB} 
%       velocity_kinematic  - Kinematic body velocity, {B}_v_{WB} 
%       filter_selector     - used to select low pass filter type
%
%
%   Author: Ross Hartley
%   Date:   11/07/2017

%% Settings
use_ekf_position = true;
use_ekf_orientation = false;
use_ekf_velocity = false;

%% Compute kinematic velocity
e = q(7:end);
e_dot = dq(7:end);

if contact(1) == 1
    pL = p_VectorNav_to_LeftToeBottom(e); % {I}_p_{IL}
    J_pL = J_VectorNav_to_LeftToeBottom(e);
    velocity_kinematic = -J_pL(1:3,:)*e_dot - Angles.skew(w)*pL(1:3,:); % {I}_v_{WI}
elseif contact(2) == 1
    pR = p_VectorNav_to_RightToeBottom(e); % {I}_p_{IR}
    J_pR = J_VectorNav_to_RightToeBottom(e);
    velocity_kinematic = -J_pR(1:3,:)*e_dot - Angles.skew(w)*pR(1:3,:); % {I}_v_{WI}
else
    velocity_kinematic = zeros(3,1);
end

%% Reconstruct State
Rbi = R_VectorNav_to_Pelvis(e)';    % R_{BI}

% Position
if use_ekf_position && ekf_enabled
    Rwi = Angles.Quaternion_to_Rotation(mu(7:10))';
    % {W}_p_{WB} =  {W}_p_{WI} +  {W}_p_{IB}
    q(1:3) = mu(1:3) + Rwi * p_VectorNav_to_Pelvis(e); 
end
 
% Orientation
if use_ekf_orientation && ekf_enabled
    Rwi = Angles.Quaternion_to_Rotation(mu(7:10))';
    Rwb = Rwi * Rbi';
    q(4:6) = Angles.Rotation_to_Euler( Rwb );
end

% Velocity
if use_ekf_velocity && ekf_enabled
    Rwi = Angles.Quaternion_to_Rotation(mu(7:10))';
    Rwb = Rwi * Rbi';
    % {W}_v_{WB} =  {W}_v_{WI} + R_{WI} * skew({I}_w_{WI}) * {I}_p_{IB}
    dq(1:3) = mu(4:6) + Rwi * Angles.skew(w) * p_VectorNav_to_Pelvis(e); 
    % {B}_v_{WB} = R_{BW} * {W}_v_{WB}
    velocity = Rwb' * dq(1:3);
    filter_selector = 1;
else
    Rwb = Angles.Euler_to_Rotation(q(4:6));
    Rwi = Rwb * Rbi;
    % {W}_v_{WB} =  R_{WI} * {I}_v_{WI} + R_{WI} * skew({I}_w_{WI}) * {I}_p_{IB}
    dq(1:3) = Rwi * velocity_kinematic + Rwi * Angles.skew(w) * p_VectorNav_to_Pelvis(e); 
    % {B}_v_{WB} = R_{BW} * {W}_v_{WB}
    velocity = Rwb' * dq(1:3);
    filter_selector = 0;
end



end

== matlab function StateEstimation/Parse Outputs/Parse_Outputs ==
  data: qwi output; wi output; ai output; q output; outputs input; dq output
function [qwi, wi, ai, q, dq] = Parse_Outputs(outputs)
%
% Frames:
%   W - Cassie World (inertial frame North-West-Up)
%   N - IMU World (inertial frame North-East-Down)
%   B - Body (cassie pelvis)
%   I - IMU (cassie vectorNav)
%   
%   Author: Ross Hartley 
%   Date:   11/06/2017
%

% Parse IMU Data from the VectorNav on Cassie
cassieOutputs = CassieOutputs;
cassieOutputs.setStructure(outputs);

% IMU Data
% VectorNav outputs quaternion as qin = [qw; qx; qy; qz]
qin = cassieOutputs.getVectorNavOrientation; qin = qin([2,3,4,1]); % Convert to [qx; qy; qz; qw] format
wi = cassieOutputs.getVectorNavAngularVelocity;      % {I}_\omega_{NI}   or   {I}_\omega_{WI}
ai = cassieOutputs.getVectorNavLinearAcceleration;   % {I}_a_{NI}        or   {I}_a_{WI}
Rni = Angles.Quaternion_to_Rotation(qin)'; % R_{NI}
Rbi = R_VectorNav_to_Pelvis(zeros(14,1))';    % R_{BI} 
Rwn = Angles.Rx(pi);                % R_{WN}
Rwi = Rwn*Rni;                      % R_{WI}
Rwb = Rwi*Rbi';                     % R_{WB}
qwi = Angles.Rotation_to_Quaternion(Rwi);
 
% Compute angular velocity of body frame:
%      {I}_\omega_{NI} = {I}_\omega_{NW} + {I}_\omega_{WB} + {I}_\omega_{BI}
%                      =        0        + {I}_\omega_{WB} +       0
%  =>  {B}_\omega_{WB} = R_{BI} * {I}_\omega_{NI}
wb = Rbi*wi; % {B}_\omega_{WB}

% Get positions
qq = Angles.Rotation_to_Euler(Rwb);
qaR = cassieOutputs.getRightLegMotorPositions;
qjR =  cassieOutputs.getRightLegJointPositions;
qaL = cassieOutputs.getLeftLegMotorPositions;
qjL =  cassieOutputs.getLeftLegJointPositions;

% Get velocities
dqq = Angles.AngularVelocity_to_EulerRates(qq, wb);
dqaR = cassieOutputs.getRightLegMotorVelocities;
dqjR =  cassieOutputs.getRightLegJointVelocities;
dqaL = cassieOutputs.getLeftLegMotorVelocities;
dqjL =  cassieOutputs.getLeftLegJointVelocities;

% Construct State Vector
q = [zeros(3,1); qq; qaL(1:3); qaL(4); qjL(1); qjL(2); qaL(5); qaR(1:3); qaR(4); qjR(1); qjR(2); qaR(5)];
dq = [zeros(3,1); dqq; dqaL(1:3); dqaL(4); dqjL(1); dqjL(2); dqaL(5); dqaR(1:3); dqaR(4); dqjR(1); dqjR(2); dqaR(5)];

end

== matlab function StateEstimation/Ground Reaction Estimator/GRF_Estimator ==
  data: q input; GRF output; contact output
function [GRF, contact] = GRF_Estimator(q)
% Estimates the ground reaction force in the body frame of the robot
%
% Fe_i = (S_i * J_i^T)^{-1} * S_i * \tau_d
%
J_pR = J_RightToeBottom([zeros(6,1); q(7:end)]);
J_pL = J_LeftToeBottom([zeros(6,1); q(7:end)]);

qs_knee_L = q(11);
qs_tarsus_L = q(10) + q(11) + q(12) - deg2rad(13);

qs_knee_R = q(18);
qs_tarsus_R = q(17) + q(18) + q(19) - deg2rad(13);

tau_L = -[1500; 1250].*[qs_knee_L + qs_tarsus_L; qs_tarsus_L];
tau_R = -[1500; 1250].*[qs_knee_R + qs_tarsus_R; qs_tarsus_R];

GRF_L = -[J_pL([1,3],11), J_pL([1,3],12)] \ tau_L;
GRF_R = -[J_pR([1,3],18), J_pR([1,3],19)] \ tau_R;
GRF = [GRF_L; GRF_R];

% Detect contact using GRF
cL = scaleFactor(GRF(2), 50, 100);
cR = scaleFactor(GRF(4), 50, 100);
contact = [cL; cR];

end
